simulink model "SimHacheur_DCM"  (R2014a)
settings: Solver=ode23tb  StartTime=0.0  StopTime=100e-3  FixedStep=11e-6  RelTol=1e-9
values from neighbouring files (symbols this model uses):
  freq = clock/steps    (= 125000)    [Init_panneau.m]
  rev_current = flipud(current)    [Init_panneau.m]
  rev_voltage = flipud(voltage)    [Init_panneau.m]
  steps = 2^resolution    (= 128)    [Init_panneau.m]
  V_Batt = 6    [Init_panneau.m]
libraries: powerlib x14, simulink x2
settings Model: Creator=hfortin  LastModifiedBy=hugo
settings DataIOCC: SignalLoggingSaveFormat=ModelDataLogs  Refine=4
settings OptimizationCC: ExpressionDepthLimit=2147483647
settings DebuggingCC: UnderspecifiedInitializationDetection=Classic  FcnCallInpInsideContextMsg=UseLocalSettings  StateNameClashWarn=warning
settings GRTTargetCC: CombineOutputUpdateFcns=off  GRTInterface=on

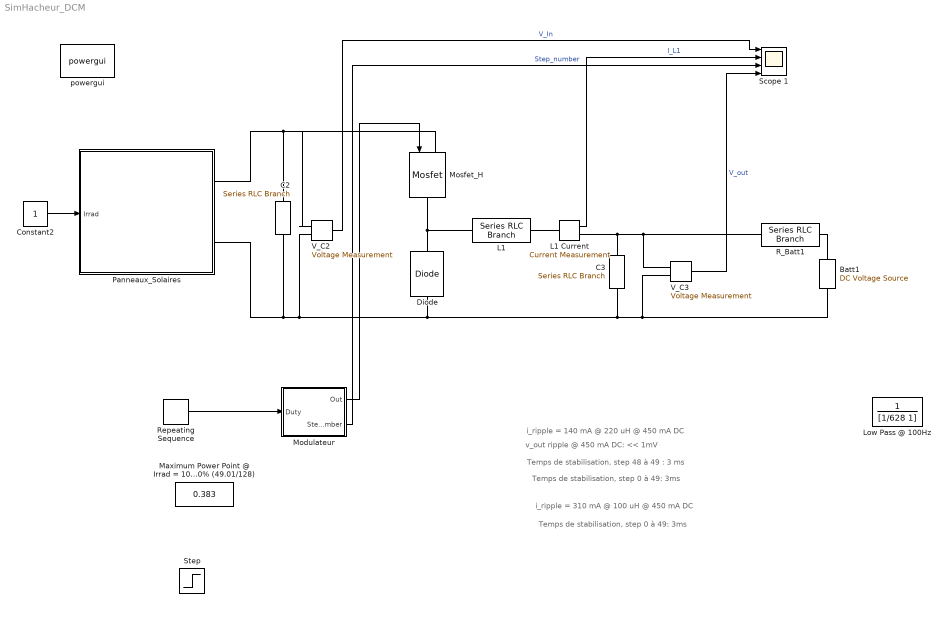
== system SimHacheur_DCM ==
  note: Temps de stabilisation, step 0 à 49: 3ms
  note: i_ripple = 310 mA @ 100 uH @ 450 mA DC
  note: v_out ripple @ 450 mA DC: << 1mV
  note: Temps de stabilisation, step 0 à 49: 3ms
  note: Temps de stabilisation, step 48 à 49 : 3 ms
  note: i_ripple = 140 mA @ 220 uH @ 450 mA DC
  Batt1 : powerlib/Electrical Sources/DC Voltage Source  Amplitude=V_Batt  Measurements=None
  C2 : powerlib/Elements/Series RLC Branch  LConnTagsString=__new0  RConnTagsString=__new0  BranchType=C  Resistance=1  Inductance=1e-3  SetiL0=off  InitialCurrent=0  Capacitance=22e-6  Setx0=on  InitialVoltage=V_Batt  Measurements=None
  C3 : powerlib/Elements/Series RLC Branch  LConnTagsString=__new0  RConnTagsString=__new0  BranchType=C  Resistance=1  Inductance=1e-3  SetiL0=off  InitialCurrent=0  Capacitance=220e-6  Setx0=on  InitialVoltage=6.022  Measurements=None
  Constant2 : Constant
  Diode : powerlib/Power Electronics/Diode  Ron=0.001  Lon=0  Vf=0.05  IC=0  UseSnubber=off  Rs=500  Cs=250e-9  Measurements=off
  L1 : powerlib/Elements/Series RLC Branch  LConnTagsString=__new0  RConnTagsString=__new0  BranchType=RL  Resistance=0.09  Inductance=100e-6  SetiL0=on  InitialCurrent=0  Capacitance=1e-6  Setx0=off  InitialVoltage=0  Measurements=None
  L1 Current : powerlib/Measurements/Current Measurement  PhasorSimulation=off  OutputType=Complex  PSBequivalent=0
  Low Pass @ 100Hz : TransferFcn  Denominator=[1/628 1]
  Maximum Power Point @ Irrad = 100% (49.01/128) : Constant  Value=0.383
  Modulateur : Subsystem
  Mosfet_H : powerlib/Power Electronics/Mosfet  Ron=RDS_on  Lon=0  Rd=0.01  Vfd=0.7  IC=0  Rs=1000000  Cs=25e-9  Measurements=off
  Panneaux_Solaires : Subsystem
  R_Batt1 : powerlib/Elements/Series RLC Branch  LConnTagsString=__new0  RConnTagsString=__new0  BranchType=R  Resistance=0.045  Inductance=1e-3  SetiL0=off  InitialCurrent=0  Capacitance=1e-6  Setx0=off  InitialVoltage=0  Measurements=None
  Repeating Sequence : simulink/Sources/Repeating Sequence  rep_seq_t=[0 0.1]  rep_seq_y=[0.33 0.42]
  Scope 1 : Scope  NumInputPorts=4
      settings: ShowLegends=on  YMin=17.06~0.38~0.0118~-5  YMax=17.24~0.53~0.0125~5
  Step : Step  Time=0.02  After=0.383  SampleTime=0
  V_C2 : powerlib/Measurements/Voltage Measurement  PhasorSimulation=off  OutputType=Complex  PSBequivalent=0
  V_C3 : powerlib/Measurements/Voltage Measurement  PhasorSimulation=off  OutputType=Complex  PSBequivalent=0
  powergui : powerlib/powergui  Priority=1  SimulationMode=Discrete  SolverType=Tustin  SampleTime=20e-9  frequency=60  SPID=off  DisableSnubberDevices=off  DisableRonSwitches=off  DisableVfSwitches=off  SwTol=0  Interpol=off  DisplayEquations=off  Ts=0  methode=off  frequencyindice=0  Pbase=100e6  ErrMax=1e-4  Iterations=50  UnitsV=kV  UnitsW=MW  FunctionMessages=off  echomessages=off  HookPort=off  EnableUseOfTLC=off  x0status=blocks  RestoreLinks=warning  ResistiveCurrentMeasurement=off  Frange=[0:2:500]  Ylog=off  Xlog=on  ShowGrid=off  save=off  variable=ZData  structure=0  ZoomFFT=on  StartTime=0.0  cycles=1  DisplayStyle=1  fundamental=60  FreqAxis=off  MaxFrequency=1000  frequencyindicesteady=1  RmsSteady=1  display=off
  wires:
  L1 Current/1 -> Scope 1/2  "I_L1"
  V_C2/1 -> Scope 1/1  "V_In"
  Constant2/1 -> Panneaux_Solaires/1(Irrad)
  Modulateur/1(Out) -> Mosfet_H/1
  Modulateur/2(Step_Number) -> Scope 1/3  "Step_number"
  V_C3/1 -> Scope 1/4  "V_out"
  Repeating Sequence/1 -> Modulateur/1(Duty)
  connections:
  Batt1/LConn1 -- Diode/LConn1 -- Panneaux_Solaires/RConn2 -- C2/RConn1 -- V_C2/LConn2 -- C3/RConn1 -- V_C3/LConn2
  L1/LConn1 -- Diode/RConn1 -- Mosfet_H/RConn1
  R_Batt1/LConn1 -- V_C3/LConn1 -- L1 Current/RConn1 -- C3/LConn1
  Batt1/RConn1 -- R_Batt1/RConn1
  C2/LConn1 -- Mosfet_H/LConn1 -- V_C2/LConn1 -- Panneaux_Solaires/RConn1
  L1 Current/LConn1 -- L1/RConn1

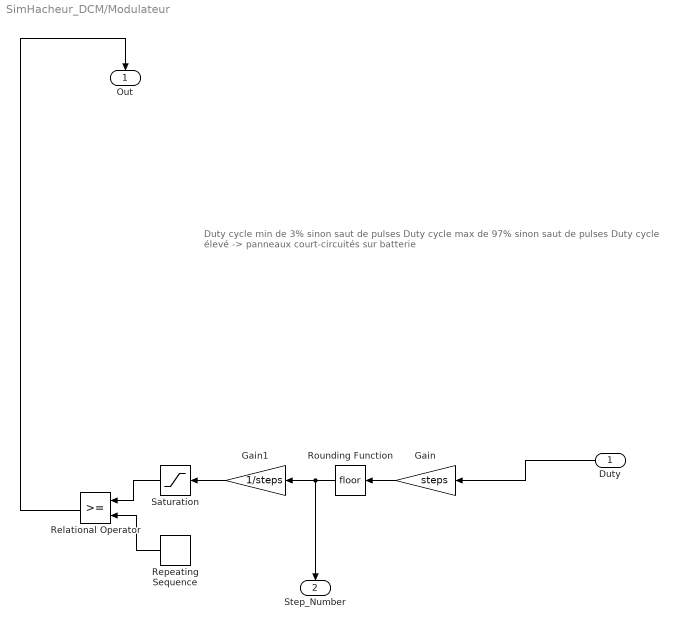
== system SimHacheur_DCM/Modulateur ==
  note: Duty cycle min de 3% sinon saut de pulses
      | Duty cycle max de 97% sinon saut de pulses
      | Duty cycle élevé -> panneaux court-circuités sur batterie
  Duty : Inport
  Gain : Gain  Gain=steps
  Gain1 : Gain  Gain=1/steps
  Relational Operator : RelationalOperator  OutDataTypeStr=boolean
  Repeating Sequence : simulink/Sources/Repeating Sequence  rep_seq_t=[0 1/freq]  rep_seq_y=[0 1]
  Rounding Function : Rounding
  Saturation : Saturate  UpperLimit=0.97  LowerLimit=0.03
  Out : Outport
  Step_Number : Outport  Port=2
  wires:
  Repeating Sequence/1 -> Relational Operator/2
  Relational Operator/1 -> Out/1
  Rounding Function/1 -> Step_Number/1, Gain1/1
  Gain/1 -> Rounding Function/1
  Duty/1 -> Gain/1
  Gain1/1 -> Saturation/1
  Saturation/1 -> Relational Operator/1

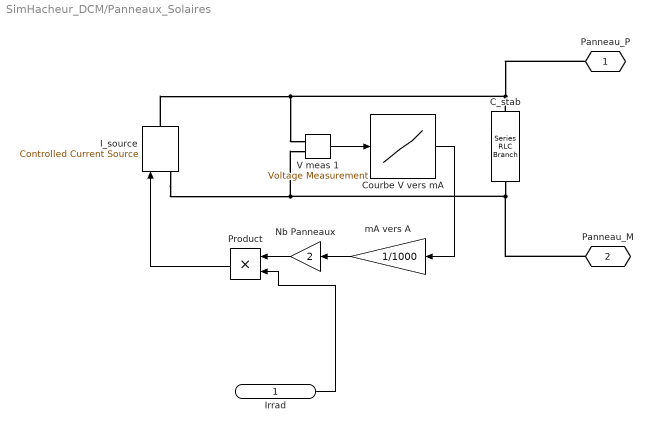
== system SimHacheur_DCM/Panneaux_Solaires ==
  Irrad : Inport
  C_stab : powerlib/Elements/Series RLC Branch  LConnTagsString=__new0  RConnTagsString=__new0  BranchType=C  Resistance=1  Inductance=1e-3  SetiL0=off  InitialCurrent=0  Capacitance=1e-9  Setx0=off  InitialVoltage=V_Batt  Measurements=None
  Courbe V vers mA : Lookup_n-D  NumberOfTableDimensions=1  BreakpointsForDimension1=rev_voltage  Table=rev_current  UseLastTableValue=on  InternalRulePriority=Speed  RndMeth=Simplest  InputSameDT=on
  I_source : powerlib/Electrical Sources/Controlled Current Source  Initialize=off  Source_Type=DC  Amplitude=0  Phase=0  Frequency=0  Measurements=None
  Nb Panneaux : Gain  Gain=2
  Product : Product
  V meas 1 : powerlib/Measurements/Voltage Measurement  PhasorSimulation=off  OutputType=Complex  PSBequivalent=0
  mA vers A : Gain  Gain=1/1000
  Panneau_P : PMIOPort  Port=1  Side=Right
  Panneau_M : PMIOPort  Port=2  Side=Right
  wires:
  Courbe V vers mA/1 -> mA vers A/1
  mA vers A/1 -> Nb Panneaux/1
  V meas 1/1 -> Courbe V vers mA/1
  Nb Panneaux/1 -> Product/1
  Product/1 -> I_source/1
  Irrad/1 -> Product/2
  connections:
  I_source/LConn1 -- V meas 1/LConn2 -- C_stab/RConn1 -- Panneau_M/RConn1
  C_stab/LConn1 -- I_source/RConn1 -- V meas 1/LConn1 -- Panneau_P/RConn1
